simulink model "Parallel_n25_D2"  (R2012b)
settings: Solver=VariableStepDiscrete  StartTime=0.0  StopTime=TotalIterations  RelTol=1e-3
values from neighbouring files (symbols this model uses):
  bp = 12    [ConfigValidate.m]
  bpSNMemory = bp    (= 12)    [ConfigValidate.m]
  IterationsOrdering = 4000    [ConfigValidate.m]
  MaxCoordDistance = (abs(max(wx) - min(wx))+abs(max(wy) - min(wy)))^2    [ConfigValidate.m]
  N_limit = 0.01    [ConfigValidate.m]
  nBits = 9    [ConfigValidate.m]
  nBitsNSmemories = (ceil(log2(TotalIterations)))    [ConfigValidate.m]
  S_limit = 1    [ConfigValidate.m]
  SourceNodes = 2000    [ConfigValidate.m]
  ts = 1    [ConfigValidate.m]
  w1 = rand(1,Neurons)    [ConfigValidate.m]
  w2 = rand(1,Neurons)    [ConfigValidate.m]
  wx = zeros(1,Neurons)    [ConfigValidate.m]
  wy = zeros(1,Neurons)    [ConfigValidate.m]
  x1 = rand(SourceNodes,1)    [ConfigValidate.m]
  x2 = rand(SourceNodes,1)    [ConfigValidate.m]
libraries: xbsIndex_r4 x1652, dspsrcs4 x2, dspstat3 x2
(part 1 of 9)
settings Model: Creator=Leonardo  LastModifiedBy=leona

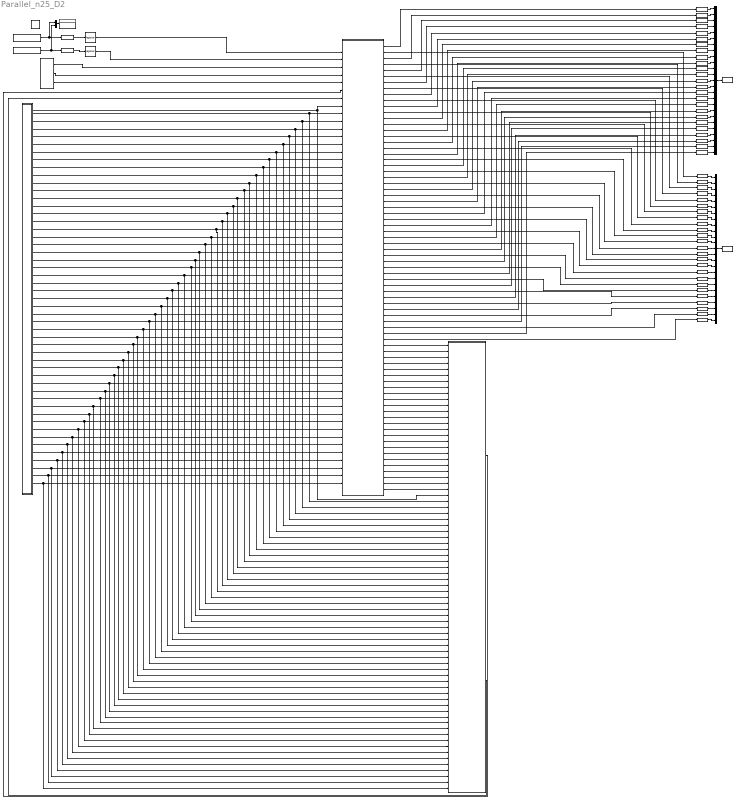
== system Parallel_n25_D2 ==
  " System Generator" : xbsIndex_r4/ System Generator  Tag=genX  xilinxfamily=virtex6  part=xc6vlx240t  speed=-1  package=ff1156  synthesis_tool=XST  clock_wrapper=Clock Enables  directory=./n25d2nt  proj_type=Project Navigator  Synth_file=XST Defaults  Impl_file=ISE Defaults  testbench=off  simulink_period=ts  sysclk_period=10  dcm_input_clock_period=10  incr_netlist=off  trim_vbits=Everywhere in SubSystem  dbl_ovrd=According to Block Masks  core_generation=According to Block Masks  run_coregen=off  deprecated_control=off  eval_field=0  block_type=sysgen
  Coordinates : Subsystem
  Display2 : Display
  Gateway Out{1..13,15..21,23..44,46..50} (47 alike) : xbsIndex_r4/Gateway Out  inherit_from_input=off  hdl_port=off  timing_constraint=None  locs_specified=off  LOCs={}  UseAsDAC=off  DACChannel='1'  block_type=gatewayout
  Gateway Out14 : xbsIndex_r4/Gateway Out  inherit_from_input=off  hdl_port=on  timing_constraint=None  locs_specified=off  LOCs={}  UseAsDAC=off  DACChannel='1'  block_type=gatewayout
  Gateway Out22 : xbsIndex_r4/Gateway Out  inherit_from_input=off  hdl_port=on  timing_constraint=None  locs_specified=off  LOCs={}  UseAsDAC=off  DACChannel='1'  block_type=gatewayout
  Gateway Out45 : xbsIndex_r4/Gateway Out  inherit_from_input=off  hdl_port=on  timing_constraint=None  locs_specified=off  LOCs={}  UseAsDAC=off  DACChannel='1'  block_type=gatewayout
  Mux3 : Mux  Inputs=2
  Mux5 : Mux  Inputs=25
  Mux6 : Mux  Inputs=25
  Neurons : Subsystem
  Signal From Workspace : dspsrcs4/Signal From Workspace  X=x1(1:SourceNodes)  Ts=ts  nsamps=1  OutputAfterFinalValue=Cyclic repetition  ignoreOrWarnInputAndFrameLengths=off
  Signal From Workspace1 : dspsrcs4/Signal From Workspace  X=x2(1:SourceNodes)  Ts=ts  nsamps=1  OutputAfterFinalValue=Cyclic repetition  ignoreOrWarnInputAndFrameLengths=off
  TimeSeries_Functions : Subsystem
  To Workspace : ToWorkspace  VariableName=w1_histH  SampleTime=ts
  To Workspace1 : ToWorkspace  VariableName=w2_histH  SampleTime=ts
  WiningNeuronFinder : Subsystem
  delay_vX11 : xbsIndex_r4/Register  init=x1(1)  rst=off  en=off  dbl_ovrd=off  block_type=register
  delay_vX12 : xbsIndex_r4/Register  init=x2(1)  rst=off  en=off  dbl_ovrd=off  block_type=register
  "vX11_in " : xbsIndex_r4/Gateway In  gui_display_data_type=Fixed-point  arith_type="Signed  (2's comp)"  n_bits=nb  bin_pt=bp  preci_type=Single  exp_width=8  frac_width=24  quantization="Round  (unbiased: +/- Inf)"  overflow=Saturate  period=ts  dbl_ovrd=off  timing_constraint=None  locs_specified=off  LOCs={}  UseAsADC=off  ADCChannel='1'  inherit_from_input=off  hdl_port=on  block_type=gatewayin
  vX12_in : xbsIndex_r4/Gateway In  gui_display_data_type=Fixed-point  arith_type="Signed  (2's comp)"  n_bits=nb  bin_pt=bp  preci_type=Single  exp_width=8  frac_width=24  quantization="Round  (unbiased: +/- Inf)"  overflow=Saturate  period=ts  dbl_ovrd=off  timing_constraint=None  locs_specified=off  LOCs={}  UseAsADC=off  ADCChannel='1'  inherit_from_input=off  hdl_port=on  block_type=gatewayin
  wires:
  Signal From Workspace/1 -> Mux3/1, "vX11_in "/1
  Signal From Workspace1/1 -> Mux3/2, vX12_in/1
  Mux3/1 -> Display2/1
  vX12_in/1 -> delay_vX12/1
  delay_vX12/1 -> Neurons/2(vX12)
  TimeSeries_Functions/1(S) -> Neurons/3(S)
  TimeSeries_Functions/2(N) -> Neurons/4(N)
  TimeSeries_Functions/3(MemControl) -> Neurons/5(memControl)
  Gateway Out1/1 -> Mux5/2
  Gateway Out14/1 -> Mux5/1
  Gateway Out10/1 -> Mux5/14
  Gateway Out8/1 -> Mux5/9
  Gateway Out17/1 -> Mux5/13
  Gateway Out6/1 -> Mux5/10
  Gateway Out4/1 -> Mux5/5
  Gateway Out2/1 -> Mux5/6
  Gateway Out13/1 -> Mux5/3
  Gateway Out15/1 -> Mux5/4
  Gateway Out9/1 -> Mux5/12
  Gateway Out18/1 -> Mux5/16
  Gateway Out7/1 -> Mux5/11
  Gateway Out16/1 -> Mux5/15
  Gateway Out3/1 -> Mux5/7
  Gateway Out5/1 -> Mux5/8
  Neurons/5(w1n3) -> Gateway Out13/1
  Neurons/7(w1n4) -> Gateway Out15/1
  Gateway Out19/1 -> Mux6/2
  Gateway Out22/1 -> Mux6/1
  Gateway Out20/1 -> Mux6/14
  Gateway Out33/1 -> Mux6/9
  Gateway Out25/1 -> Mux6/13
  Gateway Out31/1 -> Mux6/10
  Gateway Out29/1 -> Mux6/5
  Gateway Out27/1 -> Mux6/6
  Gateway Out21/1 -> Mux6/3
  Gateway Out23/1 -> Mux6/4
  Gateway Out34/1 -> Mux6/12
  Gateway Out26/1 -> Mux6/16
  Gateway Out32/1 -> Mux6/11
  Gateway Out24/1 -> Mux6/15
  Gateway Out28/1 -> Mux6/7
  Gateway Out30/1 -> Mux6/8
  Mux5/1 -> To Workspace/1
  Mux6/1 -> To Workspace1/1
  Neurons/53(dist_n3) -> WiningNeuronFinder/3(dist_k3)
  Neurons/52(dist_n2) -> WiningNeuronFinder/2(dist_k2)
  Neurons/54(dist_n4) -> WiningNeuronFinder/4(dist_k4)
  Neurons/51(dist_n1) -> WiningNeuronFinder/1(dist_k1)
  WiningNeuronFinder/1(WinningNeuron_wx) -> Neurons/6(wx_win)
  WiningNeuronFinder/2(WinningNeuron_wy) -> Neurons/7(wy_win)
  Neurons/55(dist_n5) -> WiningNeuronFinder/5(dist_k5)
  Neurons/56(dist_n6) -> WiningNeuronFinder/6(dist_k6)
  Neurons/57(dist_n7) -> WiningNeuronFinder/7(dist_k7)
  Neurons/58(dist_n8) -> WiningNeuronFinder/8(dist_k8)
  Neurons/59(dist_n9) -> WiningNeuronFinder/9(dist_k9)
  Neurons/60(dist_n10) -> WiningNeuronFinder/10(dist_k10)
  Neurons/61(dist_n11) -> WiningNeuronFinder/11(dist_k11)
  Neurons/62(dist_n12) -> WiningNeuronFinder/12(dist_k12)
  Neurons/63(dist_n13) -> WiningNeuronFinder/13(dist_k13)
  Neurons/64(dist_n14) -> WiningNeuronFinder/14(dist_k14)
  Neurons/65(dist_n15) -> WiningNeuronFinder/15(dist_k15)
  Neurons/66(dist_n16) -> WiningNeuronFinder/16(dist_k16)
  Neurons/67(dist_n17) -> WiningNeuronFinder/17(dist_k17)
  Neurons/68(dist_n18) -> WiningNeuronFinder/18(dist_k18)
  Neurons/69(dist_n19) -> WiningNeuronFinder/19(dist_k19)
  Neurons/70(dist_n20) -> WiningNeuronFinder/20(dist_k20)
  Neurons/71(dist_n21) -> WiningNeuronFinder/21(dist_k21)
  Neurons/72(dist_n22) -> WiningNeuronFinder/22(dist_k22)
  Neurons/73(dist_n23) -> WiningNeuronFinder/23(dist_k23)
  Neurons/74(dist_n24) -> WiningNeuronFinder/24(dist_k24)
  Neurons/75(dist_n25) -> WiningNeuronFinder/25(dist_k25)
  Coordinates/49(wx25) -> WiningNeuronFinder/74(wx_25), Neurons/56(wx25)
  Coordinates/48(wy24) -> WiningNeuronFinder/73(wy_24), Neurons/55(wy24)
  Coordinates/47(wx24) -> WiningNeuronFinder/72(wx_24), Neurons/54(wx24)
  Coordinates/46(wy23) -> WiningNeuronFinder/71(wy_23), Neurons/53(wy23)
  Coordinates/45(wx23) -> WiningNeuronFinder/70(wx_23), Neurons/52(wx23)
  Coordinates/44(wy22) -> WiningNeuronFinder/69(wy_22), Neurons/51(wy22)
  Coordinates/43(wx22) -> WiningNeuronFinder/68(wx_22), Neurons/50(wx22)
  Coordinates/42(wy21) -> WiningNeuronFinder/67(wy_21), Neurons/49(wy21)
  Coordinates/41(wx21) -> WiningNeuronFinder/66(wx_21), Neurons/48(wx21)
  Coordinates/40(wy20) -> WiningNeuronFinder/65(wy_20), Neurons/47(wy20)
  Coordinates/39(wx20) -> WiningNeuronFinder/64(wx_20), Neurons/46(wx20)
  Coordinates/38(wy19) -> WiningNeuronFinder/63(wy_19), Neurons/45(wy19)
  Coordinates/37(wx19) -> WiningNeuronFinder/62(wx_19), Neurons/44(wx19)
  Coordinates/36(wy18) -> WiningNeuronFinder/61(wy_18), Neurons/43(wy18)
  Coordinates/35(wx18) -> WiningNeuronFinder/60(wx_18), Neurons/42(wx18)
  Coordinates/34(wy17) -> WiningNeuronFinder/59(wy_17), Neurons/41(wy17)
  Coordinates/33(wx17) -> WiningNeuronFinder/58(wx_17), Neurons/40(wx17)
  Coordinates/32(wy16) -> WiningNeuronFinder/57(wy_16), Neurons/39(wy16)
  Coordinates/31(wx16) -> WiningNeuronFinder/56(wx_16), Neurons/38(wx16)
  Coordinates/30(wy15) -> WiningNeuronFinder/55(wy_15), Neurons/37(wy15)
  Coordinates/29(wx15) -> WiningNeuronFinder/54(wx_15), Neurons/36(wx15)
  Coordinates/28(wy14) -> WiningNeuronFinder/53(wy_14), Neurons/35(wy14)
  Coordinates/27(wx14) -> WiningNeuronFinder/52(wx_14), Neurons/34(wx14)
  Coordinates/25(wx13) -> WiningNeuronFinder/50(wx_13), Neurons/32(wx13)
  Coordinates/24(wy12) -> WiningNeuronFinder/49(wy_12), Neurons/31(wy12)
  Coordinates/23(wx12) -> WiningNeuronFinder/48(wx_12), Neurons/30(wx12)
  Coordinates/22(wy11) -> WiningNeuronFinder/47(wy_11), Neurons/29(wy11)
  Coordinates/21(wx11) -> WiningNeuronFinder/46(wx_11), Neurons/28(wx11)
  Coordinates/20(wy10) -> WiningNeuronFinder/45(wy_10), Neurons/27(wy10)
  Coordinates/19(wx10) -> WiningNeuronFinder/44(wx_10), Neurons/26(wx10)
  Coordinates/18(wy9) -> WiningNeuronFinder/43(wy_9), Neurons/25(wy9)
  Coordinates/17(wx9) -> WiningNeuronFinder/42(wx_9), Neurons/24(wx9)
  Coordinates/16(wy8) -> WiningNeuronFinder/41(wy_8), Neurons/23(wy8)
  Coordinates/15(wx8) -> WiningNeuronFinder/40(wx_8), Neurons/22(wx8)
  Coordinates/13(wx7) -> WiningNeuronFinder/38(wx_7), Neurons/20(wx7)
  Coordinates/12(wy6) -> WiningNeuronFinder/37(wy_6), Neurons/19(wy6)
  Coordinates/11(wx6) -> WiningNeuronFinder/36(wx_6), Neurons/18(wx6)
  Coordinates/10(wy5) -> WiningNeuronFinder/35(wy_5), Neurons/17(wy5)
  Coordinates/9(wx5) -> WiningNeuronFinder/34(wx_5), Neurons/16(wx5)
  Coordinates/8(wy4) -> WiningNeuronFinder/33(wy_4), Neurons/15(wy4)
  Coordinates/7(wx4) -> WiningNeuronFinder/32(wx_4), Neurons/14(wx4)
  Coordinates/6(wy3) -> WiningNeuronFinder/31(wy_3), Neurons/13(wy3)
  Coordinates/5(wx3) -> WiningNeuronFinder/30(wx_3), Neurons/12(wx3)
  Coordinates/4(wy2) -> WiningNeuronFinder/29(wy_2), Neurons/11(wy2)
  Coordinates/3(wx2) -> WiningNeuronFinder/28(wx_2), Neurons/10(wx2)
  Coordinates/2(wy1) -> WiningNeuronFinder/27(wy_1), Neurons/9(wy1)
  Coordinates/1(wx1) -> Neurons/8(wx1), WiningNeuronFinder/26(wx_1)
  Coordinates/14(wy7) -> WiningNeuronFinder/39(wy_7), Neurons/21(wy7)
  Coordinates/26(wy13) -> WiningNeuronFinder/51(wy_13), Neurons/33(wy13)
  Coordinates/50(wy25) -> WiningNeuronFinder/75(wy_25), Neurons/57(wy25)
  Neurons/9(w1n5) -> Gateway Out4/1
  Neurons/11(w1n6) -> Gateway Out2/1
  Neurons/13(w1n7) -> Gateway Out3/1
  Neurons/15(w1n8) -> Gateway Out5/1
  Neurons/17(w1n9) -> Gateway Out8/1
  Neurons/19(w1n10) -> Gateway Out6/1
  Neurons/21(w1n11) -> Gateway Out7/1
  Neurons/23(w1n12) -> Gateway Out9/1
  Neurons/25(w1n13) -> Gateway Out17/1
  Neurons/27(w1n14) -> Gateway Out10/1
  Neurons/29(w1n15) -> Gateway Out16/1
  Neurons/31(w1n16) -> Gateway Out18/1
  Gateway Out12/1 -> Mux5/24
  Gateway Out36/1 -> Mux5/25
  Gateway Out37/1 -> Mux5/17
  Gateway Out39/1 -> Mux5/20
  Gateway Out41/1 -> Mux5/21
  Gateway Out11/1 -> Mux5/23
  Gateway Out40/1 -> Mux5/18
  Gateway Out38/1 -> Mux5/19
  Gateway Out35/1 -> Mux5/22
  Neurons/33(w1n17) -> Gateway Out37/1
  Neurons/35(w1n18) -> Gateway Out40/1
  Neurons/37(w1n19) -> Gateway Out38/1
  Neurons/39(w1n20) -> Gateway Out39/1
  Neurons/41(w1n21) -> Gateway Out41/1
  Neurons/43(w1n22) -> Gateway Out35/1
  Neurons/45(w1n23) -> Gateway Out11/1
  Neurons/47(w1n24) -> Gateway Out12/1
  Neurons/49(w1n25) -> Gateway Out36/1
  Gateway Out43/1 -> Mux6/24
  Gateway Out46/1 -> Mux6/17
  Gateway Out50/1 -> Mux6/21
  Gateway Out48/1 -> Mux6/20
  Gateway Out45/1 -> Mux6/25
  Gateway Out42/1 -> Mux6/23
  Gateway Out44/1 -> Mux6/22
  Gateway Out49/1 -> Mux6/18
  Gateway Out47/1 -> Mux6/19
  Neurons/4(w2n2) -> Gateway Out19/1
  Neurons/6(w2n3) -> Gateway Out21/1
  Neurons/8(w2n4) -> Gateway Out23/1
  Neurons/10(w2n5) -> Gateway Out29/1
  Neurons/12(w2n6) -> Gateway Out27/1
  Neurons/14(w2n7) -> Gateway Out28/1
  Neurons/16(w2n8) -> Gateway Out30/1
  Neurons/18(w2n9) -> Gateway Out33/1
  Neurons/20(w2n10) -> Gateway Out31/1
  Neurons/22(w2n11) -> Gateway Out32/1
  Neurons/24(w2n12) -> Gateway Out34/1
  Neurons/26(w2n13) -> Gateway Out25/1
  Neurons/28(w2n14) -> Gateway Out20/1
  Neurons/30(w2n15) -> Gateway Out24/1
  Neurons/32(w2n16) -> Gateway Out26/1
  Neurons/34(w2n17) -> Gateway Out46/1
  Neurons/36(w2n18) -> Gateway Out49/1
  Neurons/38(w2n19) -> Gateway Out47/1
  Neurons/40(w2n20) -> Gateway Out48/1
  Neurons/42(w2n21) -> Gateway Out50/1
  Neurons/44(w2n22) -> Gateway Out44/1
  Neurons/46(w2n23) -> Gateway Out42/1
  Neurons/48(w2n24) -> Gateway Out43/1
  Neurons/50(w2n25) -> Gateway Out45/1
  "vX11_in "/1 -> delay_vX11/1
  delay_vX11/1 -> Neurons/1(vX11)
  Neurons/3(w1n2) -> Gateway Out1/1
  Neurons/1(w1n1) -> Gateway Out14/1
  Neurons/2(w2n1) -> Gateway Out22/1

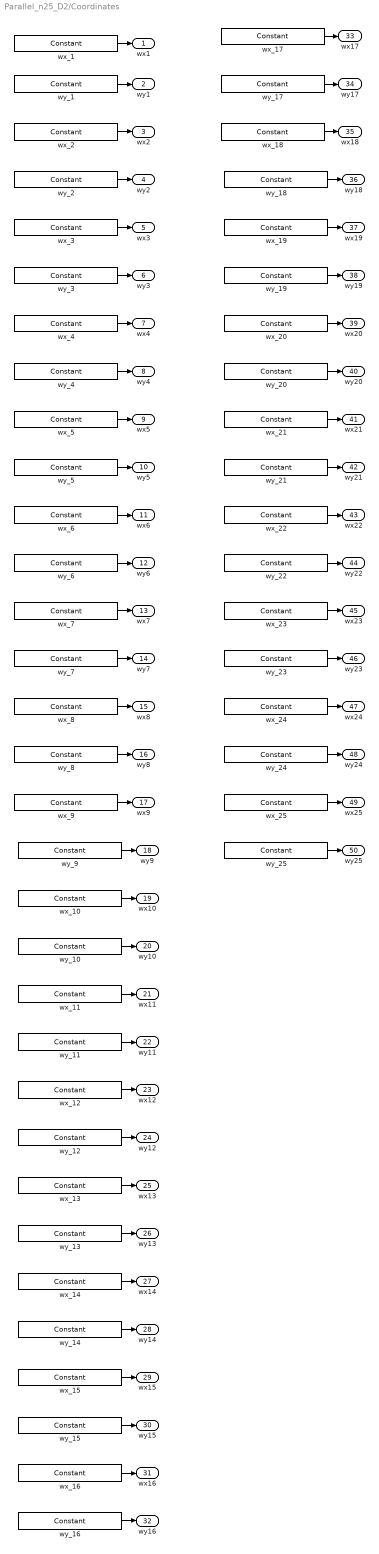
== system Parallel_n25_D2/Coordinates ==
  wx_1 : xbsIndex_r4/Constant  const=wx(1)  gui_display_data_type=Fixed-point  arith_type=Unsigned  n_bits=nbCoord  bin_pt=bpCoord  preci_type=Single  exp_width=8  frac_width=24  explicit_period=on  period=ts  equ=P=C  opselect=C  inp2=PCIN>>17  opr=+  inp1=P  carry=CIN  dbl_ovrd=off  block_type=constant
  wx_10 : xbsIndex_r4/Constant  const=wx(10)  gui_display_data_type=Fixed-point  arith_type=Unsigned  n_bits=nbCoord  bin_pt=bpCoord  preci_type=Single  exp_width=8  frac_width=24  explicit_period=on  period=ts  equ=P=C  opselect=C  inp2=PCIN>>17  opr=+  inp1=P  carry=CIN  dbl_ovrd=off  block_type=constant
  wx_11 : xbsIndex_r4/Constant  const=wx(11)  gui_display_data_type=Fixed-point  arith_type=Unsigned  n_bits=nbCoord  bin_pt=bpCoord  preci_type=Single  exp_width=8  frac_width=24  explicit_period=on  period=ts  equ=P=C  opselect=C  inp2=PCIN>>17  opr=+  inp1=P  carry=CIN  dbl_ovrd=off  block_type=constant
  wx_12 : xbsIndex_r4/Constant  const=wx(12)  gui_display_data_type=Fixed-point  arith_type=Unsigned  n_bits=nbCoord  bin_pt=bpCoord  preci_type=Single  exp_width=8  frac_width=24  explicit_period=on  period=ts  equ=P=C  opselect=C  inp2=PCIN>>17  opr=+  inp1=P  carry=CIN  dbl_ovrd=off  block_type=constant
  wx_13 : xbsIndex_r4/Constant  const=wx(13)  gui_display_data_type=Fixed-point  arith_type=Unsigned  n_bits=nbCoord  bin_pt=bpCoord  preci_type=Single  exp_width=8  frac_width=24  explicit_period=on  period=ts  equ=P=C  opselect=C  inp2=PCIN>>17  opr=+  inp1=P  carry=CIN  dbl_ovrd=off  block_type=constant
  wx_14 : xbsIndex_r4/Constant  const=wx(14)  gui_display_data_type=Fixed-point  arith_type=Unsigned  n_bits=nbCoord  bin_pt=bpCoord  preci_type=Single  exp_width=8  frac_width=24  explicit_period=on  period=ts  equ=P=C  opselect=C  inp2=PCIN>>17  opr=+  inp1=P  carry=CIN  dbl_ovrd=off  block_type=constant
  wx_15 : xbsIndex_r4/Constant  const=wx(15)  gui_display_data_type=Fixed-point  arith_type=Unsigned  n_bits=nbCoord  bin_pt=bpCoord  preci_type=Single  exp_width=8  frac_width=24  explicit_period=on  period=ts  equ=P=C  opselect=C  inp2=PCIN>>17  opr=+  inp1=P  carry=CIN  dbl_ovrd=off  block_type=constant
  wx_16 : xbsIndex_r4/Constant  const=wx(16)  gui_display_data_type=Fixed-point  arith_type=Unsigned  n_bits=nbCoord  bin_pt=bpCoord  preci_type=Single  exp_width=8  frac_width=24  explicit_period=on  period=ts  equ=P=C  opselect=C  inp2=PCIN>>17  opr=+  inp1=P  carry=CIN  dbl_ovrd=off  block_type=constant
  wx_17 : xbsIndex_r4/Constant  const=wx(17)  gui_display_data_type=Fixed-point  arith_type=Unsigned  n_bits=nbCoord  bin_pt=bpCoord  preci_type=Single  exp_width=8  frac_width=24  explicit_period=on  period=ts  equ=P=C  opselect=C  inp2=PCIN>>17  opr=+  inp1=P  carry=CIN  dbl_ovrd=off  block_type=constant
  wx_18 : xbsIndex_r4/Constant  const=wx(18)  gui_display_data_type=Fixed-point  arith_type=Unsigned  n_bits=nbCoord  bin_pt=bpCoord  preci_type=Single  exp_width=8  frac_width=24  explicit_period=on  period=ts  equ=P=C  opselect=C  inp2=PCIN>>17  opr=+  inp1=P  carry=CIN  dbl_ovrd=off  block_type=constant
  wx_19 : xbsIndex_r4/Constant  const=wx(19)  gui_display_data_type=Fixed-point  arith_type=Unsigned  n_bits=nbCoord  bin_pt=bpCoord  preci_type=Single  exp_width=8  frac_width=24  explicit_period=on  period=ts  equ=P=C  opselect=C  inp2=PCIN>>17  opr=+  inp1=P  carry=CIN  dbl_ovrd=off  block_type=constant
  wx_2 : xbsIndex_r4/Constant  const=wx(2)  gui_display_data_type=Fixed-point  arith_type=Unsigned  n_bits=nbCoord  bin_pt=bpCoord  preci_type=Single  exp_width=8  frac_width=24  explicit_period=on  period=ts  equ=P=C  opselect=C  inp2=PCIN>>17  opr=+  inp1=P  carry=CIN  dbl_ovrd=off  block_type=constant
  wx_20 : xbsIndex_r4/Constant  const=wx(20)  gui_display_data_type=Fixed-point  arith_type=Unsigned  n_bits=nbCoord  bin_pt=bpCoord  preci_type=Single  exp_width=8  frac_width=24  explicit_period=on  period=ts  equ=P=C  opselect=C  inp2=PCIN>>17  opr=+  inp1=P  carry=CIN  dbl_ovrd=off  block_type=constant
  wx_21 : xbsIndex_r4/Constant  const=wx(21)  gui_display_data_type=Fixed-point  arith_type=Unsigned  n_bits=nbCoord  bin_pt=bpCoord  preci_type=Single  exp_width=8  frac_width=24  explicit_period=on  period=ts  equ=P=C  opselect=C  inp2=PCIN>>17  opr=+  inp1=P  carry=CIN  dbl_ovrd=off  block_type=constant
  wx_22 : xbsIndex_r4/Constant  const=wx(22)  gui_display_data_type=Fixed-point  arith_type=Unsigned  n_bits=nbCoord  bin_pt=bpCoord  preci_type=Single  exp_width=8  frac_width=24  explicit_period=on  period=ts  equ=P=C  opselect=C  inp2=PCIN>>17  opr=+  inp1=P  carry=CIN  dbl_ovrd=off  block_type=constant
  wx_23 : xbsIndex_r4/Constant  const=wx(23)  gui_display_data_type=Fixed-point  arith_type=Unsigned  n_bits=nbCoord  bin_pt=bpCoord  preci_type=Single  exp_width=8  frac_width=24  explicit_period=on  period=ts  equ=P=C  opselect=C  inp2=PCIN>>17  opr=+  inp1=P  carry=CIN  dbl_ovrd=off  block_type=constant
  wx_24 : xbsIndex_r4/Constant  const=wx(24)  gui_display_data_type=Fixed-point  arith_type=Unsigned  n_bits=nbCoord  bin_pt=bpCoord  preci_type=Single  exp_width=8  frac_width=24  explicit_period=on  period=ts  equ=P=C  opselect=C  inp2=PCIN>>17  opr=+  inp1=P  carry=CIN  dbl_ovrd=off  block_type=constant
  wx_25 : xbsIndex_r4/Constant  const=wx(25)  gui_display_data_type=Fixed-point  arith_type=Unsigned  n_bits=nbCoord  bin_pt=bpCoord  preci_type=Single  exp_width=8  frac_width=24  explicit_period=on  period=ts  equ=P=C  opselect=C  inp2=PCIN>>17  opr=+  inp1=P  carry=CIN  dbl_ovrd=off  block_type=constant
  wx_3 : xbsIndex_r4/Constant  const=wx(3)  gui_display_data_type=Fixed-point  arith_type=Unsigned  n_bits=nbCoord  bin_pt=bpCoord  preci_type=Single  exp_width=8  frac_width=24  explicit_period=on  period=ts  equ=P=C  opselect=C  inp2=PCIN>>17  opr=+  inp1=P  carry=CIN  dbl_ovrd=off  block_type=constant
  wx_4 : xbsIndex_r4/Constant  const=wx(4)  gui_display_data_type=Fixed-point  arith_type=Unsigned  n_bits=nbCoord  bin_pt=bpCoord  preci_type=Single  exp_width=8  frac_width=24  explicit_period=on  period=ts  equ=P=C  opselect=C  inp2=PCIN>>17  opr=+  inp1=P  carry=CIN  dbl_ovrd=off  block_type=constant
  wx_5 : xbsIndex_r4/Constant  const=wx(5)  gui_display_data_type=Fixed-point  arith_type=Unsigned  n_bits=nbCoord  bin_pt=bpCoord  preci_type=Single  exp_width=8  frac_width=24  explicit_period=on  period=ts  equ=P=C  opselect=C  inp2=PCIN>>17  opr=+  inp1=P  carry=CIN  dbl_ovrd=off  block_type=constant
  wx_6 : xbsIndex_r4/Constant  const=wx(6)  gui_display_data_type=Fixed-point  arith_type=Unsigned  n_bits=nbCoord  bin_pt=bpCoord  preci_type=Single  exp_width=8  frac_width=24  explicit_period=on  period=ts  equ=P=C  opselect=C  inp2=PCIN>>17  opr=+  inp1=P  carry=CIN  dbl_ovrd=off  block_type=constant
  wx_7 : xbsIndex_r4/Constant  const=wx(7)  gui_display_data_type=Fixed-point  arith_type=Unsigned  n_bits=nbCoord  bin_pt=bpCoord  preci_type=Single  exp_width=8  frac_width=24  explicit_period=on  period=ts  equ=P=C  opselect=C  inp2=PCIN>>17  opr=+  inp1=P  carry=CIN  dbl_ovrd=off  block_type=constant
  wx_8 : xbsIndex_r4/Constant  const=wx(8)  gui_display_data_type=Fixed-point  arith_type=Unsigned  n_bits=nbCoord  bin_pt=bpCoord  preci_type=Single  exp_width=8  frac_width=24  explicit_period=on  period=ts  equ=P=C  opselect=C  inp2=PCIN>>17  opr=+  inp1=P  carry=CIN  dbl_ovrd=off  block_type=constant
  wx_9 : xbsIndex_r4/Constant  const=wx(9)  gui_display_data_type=Fixed-point  arith_type=Unsigned  n_bits=nbCoord  bin_pt=bpCoord  preci_type=Single  exp_width=8  frac_width=24  explicit_period=on  period=ts  equ=P=C  opselect=C  inp2=PCIN>>17  opr=+  inp1=P  carry=CIN  dbl_ovrd=off  block_type=constant
  wy_1 : xbsIndex_r4/Constant  const=wy(1)  gui_display_data_type=Fixed-point  arith_type=Unsigned  n_bits=nbCoord  bin_pt=bpCoord  preci_type=Single  exp_width=8  frac_width=24  explicit_period=on  period=ts  equ=P=C  opselect=C  inp2=PCIN>>17  opr=+  inp1=P  carry=CIN  dbl_ovrd=off  block_type=constant
  wy_10 : xbsIndex_r4/Constant  const=wy(10)  gui_display_data_type=Fixed-point  arith_type=Unsigned  n_bits=nbCoord  bin_pt=bpCoord  preci_type=Single  exp_width=8  frac_width=24  explicit_period=on  period=ts  equ=P=C  opselect=C  inp2=PCIN>>17  opr=+  inp1=P  carry=CIN  dbl_ovrd=off  block_type=constant
  wy_11 : xbsIndex_r4/Constant  const=wy(11)  gui_display_data_type=Fixed-point  arith_type=Unsigned  n_bits=nbCoord  bin_pt=bpCoord  preci_type=Single  exp_width=8  frac_width=24  explicit_period=on  period=ts  equ=P=C  opselect=C  inp2=PCIN>>17  opr=+  inp1=P  carry=CIN  dbl_ovrd=off  block_type=constant
  wy_12 : xbsIndex_r4/Constant  const=wy(12)  gui_display_data_type=Fixed-point  arith_type=Unsigned  n_bits=nbCoord  bin_pt=bpCoord  preci_type=Single  exp_width=8  frac_width=24  explicit_period=on  period=ts  equ=P=C  opselect=C  inp2=PCIN>>17  opr=+  inp1=P  carry=CIN  dbl_ovrd=off  block_type=constant
  wy_13 : xbsIndex_r4/Constant  const=wy(13)  gui_display_data_type=Fixed-point  arith_type=Unsigned  n_bits=nbCoord  bin_pt=bpCoord  preci_type=Single  exp_width=8  frac_width=24  explicit_period=on  period=ts  equ=P=C  opselect=C  inp2=PCIN>>17  opr=+  inp1=P  carry=CIN  dbl_ovrd=off  block_type=constant
  wy_14 : xbsIndex_r4/Constant  const=wy(14)  gui_display_data_type=Fixed-point  arith_type=Unsigned  n_bits=nbCoord  bin_pt=bpCoord  preci_type=Single  exp_width=8  frac_width=24  explicit_period=on  period=ts  equ=P=C  opselect=C  inp2=PCIN>>17  opr=+  inp1=P  carry=CIN  dbl_ovrd=off  block_type=constant
  wy_15 : xbsIndex_r4/Constant  const=wy(15)  gui_display_data_type=Fixed-point  arith_type=Unsigned  n_bits=nbCoord  bin_pt=bpCoord  preci_type=Single  exp_width=8  frac_width=24  explicit_period=on  period=ts  equ=P=C  opselect=C  inp2=PCIN>>17  opr=+  inp1=P  carry=CIN  dbl_ovrd=off  block_type=constant
  wy_16 : xbsIndex_r4/Constant  const=wy(16)  gui_display_data_type=Fixed-point  arith_type=Unsigned  n_bits=nbCoord  bin_pt=bpCoord  preci_type=Single  exp_width=8  frac_width=24  explicit_period=on  period=ts  equ=P=C  opselect=C  inp2=PCIN>>17  opr=+  inp1=P  carry=CIN  dbl_ovrd=off  block_type=constant
  wy_17 : xbsIndex_r4/Constant  const=wy(17)  gui_display_data_type=Fixed-point  arith_type=Unsigned  n_bits=nbCoord  bin_pt=bpCoord  preci_type=Single  exp_width=8  frac_width=24  explicit_period=on  period=ts  equ=P=C  opselect=C  inp2=PCIN>>17  opr=+  inp1=P  carry=CIN  dbl_ovrd=off  block_type=constant
  wy_18 : xbsIndex_r4/Constant  const=wy(18)  gui_display_data_type=Fixed-point  arith_type=Unsigned  n_bits=nbCoord  bin_pt=bpCoord  preci_type=Single  exp_width=8  frac_width=24  explicit_period=on  period=ts  equ=P=C  opselect=C  inp2=PCIN>>17  opr=+  inp1=P  carry=CIN  dbl_ovrd=off  block_type=constant
  wy_19 : xbsIndex_r4/Constant  const=wy(19)  gui_display_data_type=Fixed-point  arith_type=Unsigned  n_bits=nbCoord  bin_pt=bpCoord  preci_type=Single  exp_width=8  frac_width=24  explicit_period=on  period=ts  equ=P=C  opselect=C  inp2=PCIN>>17  opr=+  inp1=P  carry=CIN  dbl_ovrd=off  block_type=constant
  wy_2 : xbsIndex_r4/Constant  const=wy(2)  gui_display_data_type=Fixed-point  arith_type=Unsigned  n_bits=nbCoord  bin_pt=bpCoord  preci_type=Single  exp_width=8  frac_width=24  explicit_period=on  period=ts  equ=P=C  opselect=C  inp2=PCIN>>17  opr=+  inp1=P  carry=CIN  dbl_ovrd=off  block_type=constant
  wy_20 : xbsIndex_r4/Constant  const=wy(20)  gui_display_data_type=Fixed-point  arith_type=Unsigned  n_bits=nbCoord  bin_pt=bpCoord  preci_type=Single  exp_width=8  frac_width=24  explicit_period=on  period=ts  equ=P=C  opselect=C  inp2=PCIN>>17  opr=+  inp1=P  carry=CIN  dbl_ovrd=off  block_type=constant
  wy_21 : xbsIndex_r4/Constant  const=wy(21)  gui_display_data_type=Fixed-point  arith_type=Unsigned  n_bits=nbCoord  bin_pt=bpCoord  preci_type=Single  exp_width=8  frac_width=24  explicit_period=on  period=ts  equ=P=C  opselect=C  inp2=PCIN>>17  opr=+  inp1=P  carry=CIN  dbl_ovrd=off  block_type=constant
  wy_22 : xbsIndex_r4/Constant  const=wy(22)  gui_display_data_type=Fixed-point  arith_type=Unsigned  n_bits=nbCoord  bin_pt=bpCoord  preci_type=Single  exp_width=8  frac_width=24  explicit_period=on  period=ts  equ=P=C  opselect=C  inp2=PCIN>>17  opr=+  inp1=P  carry=CIN  dbl_ovrd=off  block_type=constant
  wy_23 : xbsIndex_r4/Constant  const=wy(23)  gui_display_data_type=Fixed-point  arith_type=Unsigned  n_bits=nbCoord  bin_pt=bpCoord  preci_type=Single  exp_width=8  frac_width=24  explicit_period=on  period=ts  equ=P=C  opselect=C  inp2=PCIN>>17  opr=+  inp1=P  carry=CIN  dbl_ovrd=off  block_type=constant
  wy_24 : xbsIndex_r4/Constant  const=wy(24)  gui_display_data_type=Fixed-point  arith_type=Unsigned  n_bits=nbCoord  bin_pt=bpCoord  preci_type=Single  exp_width=8  frac_width=24  explicit_period=on  period=ts  equ=P=C  opselect=C  inp2=PCIN>>17  opr=+  inp1=P  carry=CIN  dbl_ovrd=off  block_type=constant
  wy_25 : xbsIndex_r4/Constant  const=wy(25)  gui_display_data_type=Fixed-point  arith_type=Unsigned  n_bits=nbCoord  bin_pt=bpCoord  preci_type=Single  exp_width=8  frac_width=24  explicit_period=on  period=ts  equ=P=C  opselect=C  inp2=PCIN>>17  opr=+  inp1=P  carry=CIN  dbl_ovrd=off  block_type=constant
  wy_3 : xbsIndex_r4/Constant  const=wy(3)  gui_display_data_type=Fixed-point  arith_type=Unsigned  n_bits=nbCoord  bin_pt=bpCoord  preci_type=Single  exp_width=8  frac_width=24  explicit_period=on  period=ts  equ=P=C  opselect=C  inp2=PCIN>>17  opr=+  inp1=P  carry=CIN  dbl_ovrd=off  block_type=constant
  wy_4 : xbsIndex_r4/Constant  const=wy(4)  gui_display_data_type=Fixed-point  arith_type=Unsigned  n_bits=nbCoord  bin_pt=bpCoord  preci_type=Single  exp_width=8  frac_width=24  explicit_period=on  period=ts  equ=P=C  opselect=C  inp2=PCIN>>17  opr=+  inp1=P  carry=CIN  dbl_ovrd=off  block_type=constant
  wy_5 : xbsIndex_r4/Constant  const=wy(5)  gui_display_data_type=Fixed-point  arith_type=Unsigned  n_bits=nbCoord  bin_pt=bpCoord  preci_type=Single  exp_width=8  frac_width=24  explicit_period=on  period=ts  equ=P=C  opselect=C  inp2=PCIN>>17  opr=+  inp1=P  carry=CIN  dbl_ovrd=off  block_type=constant
  wy_6 : xbsIndex_r4/Constant  const=wy(6)  gui_display_data_type=Fixed-point  arith_type=Unsigned  n_bits=nbCoord  bin_pt=bpCoord  preci_type=Single  exp_width=8  frac_width=24  explicit_period=on  period=ts  equ=P=C  opselect=C  inp2=PCIN>>17  opr=+  inp1=P  carry=CIN  dbl_ovrd=off  block_type=constant
  wy_7 : xbsIndex_r4/Constant  const=wy(7)  gui_display_data_type=Fixed-point  arith_type=Unsigned  n_bits=nbCoord  bin_pt=bpCoord  preci_type=Single  exp_width=8  frac_width=24  explicit_period=on  period=ts  equ=P=C  opselect=C  inp2=PCIN>>17  opr=+  inp1=P  carry=CIN  dbl_ovrd=off  block_type=constant
  wy_8 : xbsIndex_r4/Constant  const=wy(8)  gui_display_data_type=Fixed-point  arith_type=Unsigned  n_bits=nbCoord  bin_pt=bpCoord  preci_type=Single  exp_width=8  frac_width=24  explicit_period=on  period=ts  equ=P=C  opselect=C  inp2=PCIN>>17  opr=+  inp1=P  carry=CIN  dbl_ovrd=off  block_type=constant
  wy_9 : xbsIndex_r4/Constant  const=wy(9)  gui_display_data_type=Fixed-point  arith_type=Unsigned  n_bits=nbCoord  bin_pt=bpCoord  preci_type=Single  exp_width=8  frac_width=24  explicit_period=on  period=ts  equ=P=C  opselect=C  inp2=PCIN>>17  opr=+  inp1=P  carry=CIN  dbl_ovrd=off  block_type=constant
  wx1 : Outport
  wy1 : Outport  Port=2
  wx2 : Outport  Port=3
  wy2 : Outport  Port=4
  wx3 : Outport  Port=5
  wy3 : Outport  Port=6
  wx4 : Outport  Port=7
  wy4 : Outport  Port=8
  wx5 : Outport  Port=9
  wy5 : Outport  Port=10
  wx6 : Outport  Port=11
  wy6 : Outport  Port=12
  wx7 : Outport  Port=13
  wy7 : Outport  Port=14
  wx8 : Outport  Port=15
  wy8 : Outport  Port=16
  wx9 : Outport  Port=17
  wy9 : Outport  Port=18
  wx10 : Outport  Port=19
  wy10 : Outport  Port=20
  wx11 : Outport  Port=21
  wy11 : Outport  Port=22
  wx12 : Outport  Port=23
  wy12 : Outport  Port=24
  wx13 : Outport  Port=25
  wy13 : Outport  Port=26
  wx14 : Outport  Port=27
  wy14 : Outport  Port=28
  wx15 : Outport  Port=29
  wy15 : Outport  Port=30
  wx16 : Outport  Port=31
  wy16 : Outport  Port=32
  wx17 : Outport  Port=33
  wy17 : Outport  Port=34
  wx18 : Outport  Port=35
  wy18 : Outport  Port=36
  wx19 : Outport  Port=37
  wy19 : Outport  Port=38
  wx20 : Outport  Port=39
  wy20 : Outport  Port=40
  wx21 : Outport  Port=41
  wy21 : Outport  Port=42
  wx22 : Outport  Port=43
  wy22 : Outport  Port=44
  wx23 : Outport  Port=45
  wy23 : Outport  Port=46
  wx24 : Outport  Port=47
  wy24 : Outport  Port=48
  wx25 : Outport  Port=49
  wy25 : Outport  Port=50
  wires:
  wy_2/1 -> wy2/1
  wy_16/1 -> wy16/1
  wx_9/1 -> wx9/1
  wy_3/1 -> wy3/1
  wx_3/1 -> wx3/1
  wy_5/1 -> wy5/1
  wx_2/1 -> wx2/1
  wx_12/1 -> wx12/1
  wy_6/1 -> wy6/1
  wx_11/1 -> wx11/1
  wy_11/1 -> wy11/1
  wy_14/1 -> wy14/1
  wy_8/1 -> wy8/1
  wy_7/1 -> wy7/1
  wx_8/1 -> wx8/1
  wx_5/1 -> wx5/1
  wx_4/1 -> wx4/1
  wx_7/1 -> wx7/1
  wx_15/1 -> wx15/1
  wy_1/1 -> wy1/1
  wy_4/1 -> wy4/1
  wx_16/1 -> wx16/1
  wx_6/1 -> wx6/1
  wy_13/1 -> wy13/1
  wx_14/1 -> wx14/1
  wy_15/1 -> wy15/1
  wx_10/1 -> wx10/1
  wy_10/1 -> wy10/1
  wx_13/1 -> wx13/1
  wy_9/1 -> wy9/1
  wy_12/1 -> wy12/1
  wy_25/1 -> wy25/1
  wx_18/1 -> wx18/1
  wx_21/1 -> wx21/1
  wx_20/1 -> wx20/1
  wy_20/1 -> wy20/1
  wy_23/1 -> wy23/1
  wy_17/1 -> wy17/1
  wx_17/1 -> wx17/1
  wx_24/1 -> wx24/1
  wx_25/1 -> wx25/1
  wy_22/1 -> wy22/1
  wx_23/1 -> wx23/1
  wy_24/1 -> wy24/1
  wx_19/1 -> wx19/1
  wy_19/1 -> wy19/1
  wx_22/1 -> wx22/1
  wy_18/1 -> wy18/1
  wy_21/1 -> wy21/1
  wx_1/1 -> wx1/1

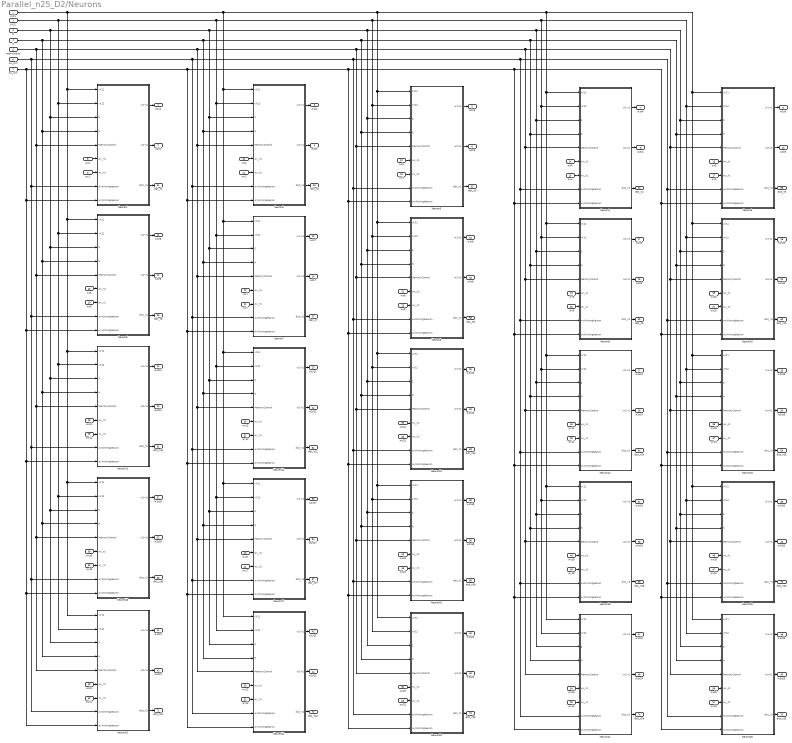
== system Parallel_n25_D2/Neurons ==
  vX11 : Inport
  vX12 : Inport  Port=2
  S : Inport  Port=3
  N : Inport  Port=4
  memControl : Inport  Port=5
  wx_win : Inport  Port=6
  wy_win : Inport  Port=7
  wx1 : Inport  Port=8
  wy1 : Inport  Port=9
  wx2 : Inport  Port=10
  wy2 : Inport  Port=11
  wx3 : Inport  Port=12
  wy3 : Inport  Port=13
  wx4 : Inport  Port=14
  wy4 : Inport  Port=15
  wx5 : Inport  Port=16
  wy5 : Inport  Port=17
  wx6 : Inport  Port=18
  wy6 : Inport  Port=19
  wx7 : Inport  Port=20
  wy7 : Inport  Port=21
  wx8 : Inport  Port=22
  wy8 : Inport  Port=23
  wx9 : Inport  Port=24
  wy9 : Inport  Port=25
  wx10 : Inport  Port=26
  wy10 : Inport  Port=27
  wx11 : Inport  Port=28
  wy11 : Inport  Port=29
  wx12 : Inport  Port=30
  wy12 : Inport  Port=31
  wx13 : Inport  Port=32
  wy13 : Inport  Port=33
  wx14 : Inport  Port=34
  wy14 : Inport  Port=35
  wx15 : Inport  Port=36
  wy15 : Inport  Port=37
  wx16 : Inport  Port=38
  wy16 : Inport  Port=39
  wx17 : Inport  Port=40
  wy17 : Inport  Port=41
  wx18 : Inport  Port=42
  wy18 : Inport  Port=43
  wx19 : Inport  Port=44
  wy19 : Inport  Port=45
  wx20 : Inport  Port=46
  wy20 : Inport  Port=47
  wx21 : Inport  Port=48
  wy21 : Inport  Port=49
  wx22 : Inport  Port=50
  wy22 : Inport  Port=51
  wx23 : Inport  Port=52
  wy23 : Inport  Port=53
  wx24 : Inport  Port=54
  wy24 : Inport  Port=55
  wx25 : Inport  Port=56
  wy25 : Inport  Port=57
  Neuron1 : Subsystem
  Neuron10 : Subsystem
  Neuron11 : Subsystem
  Neuron12 : Subsystem
  Neuron13 : Subsystem
  Neuron14 : Subsystem
  Neuron15 : Subsystem
  Neuron16 : Subsystem
  Neuron17 : Subsystem
  Neuron18 : Subsystem
  Neuron19 : Subsystem
  Neuron2 : Subsystem
  Neuron20 : Subsystem
  Neuron21 : Subsystem
  Neuron22 : Subsystem
  Neuron23 : Subsystem
  Neuron24 : Subsystem
  Neuron25 : Subsystem
  Neuron3 : Subsystem
  Neuron4 : Subsystem
  Neuron5 : Subsystem
  Neuron6 : Subsystem
  Neuron7 : Subsystem
  Neuron8 : Subsystem
  Neuron9 : Subsystem
  w1n1 : Outport
  w2n1 : Outport  Port=2
  w1n2 : Outport  Port=3
  w2n2 : Outport  Port=4
  w1n3 : Outport  Port=5
  w2n3 : Outport  Port=6
  w1n4 : Outport  Port=7
  w2n4 : Outport  Port=8
  w1n5 : Outport  Port=9
  w2n5 : Outport  Port=10
  w1n6 : Outport  Port=11
  w2n6 : Outport  Port=12
  w1n7 : Outport  Port=13
  w2n7 : Outport  Port=14
  w1n8 : Outport  Port=15
  w2n8 : Outport  Port=16
  w1n9 : Outport  Port=17
  w2n9 : Outport  Port=18
  w1n10 : Outport  Port=19
  w2n10 : Outport  Port=20
  w1n11 : Outport  Port=21
  w2n11 : Outport  Port=22
  w1n12 : Outport  Port=23
  w2n12 : Outport  Port=24
  w1n13 : Outport  Port=25
  w2n13 : Outport  Port=26
  w1n14 : Outport  Port=27
  w2n14 : Outport  Port=28
  w1n15 : Outport  Port=29
  w2n15 : Outport  Port=30
  w1n16 : Outport  Port=31
  w2n16 : Outport  Port=32
  w1n17 : Outport  Port=33
  w2n17 : Outport  Port=34
  w1n18 : Outport  Port=35
  w2n18 : Outport  Port=36
  w1n19 : Outport  Port=37
  w2n19 : Outport  Port=38
  w1n20 : Outport  Port=39
  w2n20 : Outport  Port=40
  w1n21 : Outport  Port=41
  w2n21 : Outport  Port=42
  w1n22 : Outport  Port=43
  w2n22 : Outport  Port=44
  w1n23 : Outport  Port=45
  w2n23 : Outport  Port=46
  w1n24 : Outport  Port=47
  w2n24 : Outport  Port=48
  w1n25 : Outport  Port=49
  w2n25 : Outport  Port=50
  dist_n1 : Outport  Port=51
  dist_n2 : Outport  Port=52
  dist_n3 : Outport  Port=53
  dist_n4 : Outport  Port=54
  dist_n5 : Outport  Port=55
  dist_n6 : Outport  Port=56
  dist_n7 : Outport  Port=57
  dist_n8 : Outport  Port=58
  dist_n9 : Outport  Port=59
  dist_n10 : Outport  Port=60
  dist_n11 : Outport  Port=61
  dist_n12 : Outport  Port=62
  dist_n13 : Outport  Port=63
  dist_n14 : Outport  Port=64
  dist_n15 : Outport  Port=65
  dist_n16 : Outport  Port=66
  dist_n17 : Outport  Port=67
  dist_n18 : Outport  Port=68
  dist_n19 : Outport  Port=69
  dist_n20 : Outport  Port=70
  dist_n21 : Outport  Port=71
  dist_n22 : Outport  Port=72
  dist_n23 : Outport  Port=73
  dist_n24 : Outport  Port=74
  dist_n25 : Outport  Port=75
  wires:
  wy1/1 -> Neuron1/7(wy_n1)
  Neuron2/1(w1-n1) -> w1n2/1
  Neuron3/2(w2-n1) -> w2n3/1
  Neuron1/1(w1-n1) -> w1n1/1
  Neuron2/2(w2-n1) -> w2n2/1
  Neuron1/2(w2-n1) -> w2n1/1
  wy3/1 -> Neuron3/7(wy_n1)
  wy2/1 -> Neuron2/7(wy_n1)
  Neuron3/1(w1-n1) -> w1n3/1
  wx3/1 -> Neuron3/6(wx_n1)
  wx2/1 -> Neuron2/6(wx_n1)
  Neuron4/2(w2-n1) -> w2n4/1
  wy4/1 -> Neuron4/7(wy_n1)
  wx4/1 -> Neuron4/6(wx_n1)
  Neuron4/1(w1-n1) -> w1n4/1
  Neuron1/3(dist_n1) -> dist_n1/1
  Neuron2/3(dist_n1) -> dist_n2/1
  Neuron3/3(dist_n1) -> dist_n3/1
  Neuron4/3(dist_n1) -> dist_n4/1
  memControl/1 -> Neuron5/5(MemoryControl), Neuron25/5(MemoryControl), Neuron20/5(MemoryControl), Neuron15/5(MemoryControl), Neuron10/5(MemoryControl), Neuron9/5(MemoryControl), Neuron24/5(MemoryControl), Neuron19/5(MemoryControl), Neuron14/5(MemoryControl), Neuron4/5(MemoryControl), Neuron23/5(MemoryControl), Neuron18/5(MemoryControl), Neuron13/5(MemoryControl), Neuron8/5(MemoryControl), Neuron3/5(MemoryControl), Neuron22/5(MemoryControl), Neuron17/5(MemoryControl), Neuron12/5(MemoryControl), Neuron7/5(MemoryControl), Neuron2/5(MemoryControl), Neuron21/5(MemoryControl), Neuron16/5(MemoryControl), Neuron11/5(MemoryControl), Neuron6/5(MemoryControl), Neuron1/5(MemoryControl)
  S/1 -> Neuron25/3(S), Neuron20/3(S), Neuron15/3(S), Neuron10/3(S), Neuron5/3(S), Neuron24/3(S), Neuron19/3(S), Neuron14/3(S), Neuron9/3(S), Neuron4/3(S), Neuron13/3(S), Neuron23/3(S), Neuron18/3(S), Neuron8/3(S), Neuron3/3(S), Neuron7/3(S), Neuron22/3(S), Neuron17/3(S), Neuron12/3(S), Neuron2/3(S), Neuron21/3(S), Neuron16/3(S), Neuron11/3(S), Neuron6/3(S), Neuron1/3(S)
  N/1 -> Neuron25/4(N), Neuron20/4(N), Neuron15/4(N), Neuron10/4(N), Neuron5/4(N), Neuron24/4(N), Neuron19/4(N), Neuron14/4(N), Neuron9/4(N), Neuron4/4(N), Neuron23/4(N), Neuron18/4(N), Neuron13/4(N), Neuron8/4(N), Neuron3/4(N), Neuron22/4(N), Neuron17/4(N), Neuron12/4(N), Neuron7/4(N), Neuron2/4(N), Neuron21/4(N), Neuron16/4(N), Neuron11/4(N), Neuron6/4(N), Neuron1/4(N)
  vX12/1 -> Neuron25/2(vX12), Neuron20/2(vX12), Neuron15/2(vX12), Neuron10/2(vX12), Neuron5/2(vX12), Neuron24/2(vX12), Neuron19/2(vX12), Neuron14/2(vX12), Neuron9/2(vX12), Neuron4/2(vX12), Neuron23/2(vX12), Neuron18/2(vX12), Neuron13/2(vX12), Neuron8/2(vX12), Neuron3/2(vX12), Neuron12/2(vX12), Neuron22/2(vX12), Neuron17/2(vX12), Neuron7/2(vX12), Neuron2/2(vX12), Neuron21/2(vX12), Neuron16/2(vX12), Neuron11/2(vX12), Neuron6/2(vX12), Neuron1/2(vX12)
  vX11/1 -> Neuron4/1(vX11), Neuron24/1(vX11), Neuron19/1(vX11), Neuron14/1(vX11), Neuron9/1(vX11), Neuron25/1(vX11), Neuron20/1(vX11), Neuron15/1(vX11), Neuron10/1(vX11), Neuron5/1(vX11), Neuron23/1(vX11), Neuron18/1(vX11), Neuron13/1(vX11), Neuron8/1(vX11), Neuron3/1(vX11), Neuron22/1(vX11), Neuron17/1(vX11), Neuron12/1(vX11), Neuron7/1(vX11), Neuron2/1(vX11), Neuron1/1(vX11), Neuron21/1(vX11), Neuron16/1(vX11), Neuron11/1(vX11), Neuron6/1(vX11)
  wx_win/1 -> Neuron24/8(wxWinningNeuron), Neuron19/8(wxWinningNeuron), Neuron14/8(wxWinningNeuron), Neuron9/8(wxWinningNeuron), Neuron4/8(wxWinningNeuron), Neuron25/8(wxWinningNeuron), Neuron20/8(wxWinningNeuron), Neuron15/8(wxWinningNeuron), Neuron10/8(wxWinningNeuron), Neuron5/8(wxWinningNeuron), Neuron23/8(wxWinningNeuron), Neuron18/8(wxWinningNeuron), Neuron13/8(wxWinningNeuron), Neuron8/8(wxWinningNeuron), Neuron3/8(wxWinningNeuron), Neuron22/8(wxWinningNeuron), Neuron17/8(wxWinningNeuron), Neuron12/8(wxWinningNeuron), Neuron7/8(wxWinningNeuron), Neuron2/8(wxWinningNeuron), Neuron21/8(wxWinningNeuron), Neuron16/8(wxWinningNeuron), Neuron11/8(wxWinningNeuron), Neuron6/8(wxWinningNeuron), Neuron1/8(wxWinningNeuron)
  wy_win/1 -> Neuron21/9(wyWinningNeuron), Neuron16/9(wyWinningNeuron), Neuron11/9(wyWinningNeuron), Neuron6/9(wyWinningNeuron), Neuron1/9(wyWinningNeuron), Neuron22/9(wyWinningNeuron), Neuron17/9(wyWinningNeuron), Neuron12/9(wyWinningNeuron), Neuron7/9(wyWinningNeuron), Neuron2/9(wyWinningNeuron), Neuron23/9(wyWinningNeuron), Neuron18/9(wyWinningNeuron), Neuron13/9(wyWinningNeuron), Neuron8/9(wyWinningNeuron), Neuron3/9(wyWinningNeuron), Neuron24/9(wyWinningNeuron), Neuron19/9(wyWinningNeuron), Neuron14/9(wyWinningNeuron), Neuron9/9(wyWinningNeuron), Neuron4/9(wyWinningNeuron), Neuron25/9(wyWinningNeuron), Neuron20/9(wyWinningNeuron), Neuron15/9(wyWinningNeuron), Neuron10/9(wyWinningNeuron), Neuron5/9(wyWinningNeuron)
  wy5/1 -> Neuron5/7(wy_n1)
  wx5/1 -> Neuron5/6(wx_n1)
  wy6/1 -> Neuron6/7(wy_n1)
  wx6/1 -> Neuron6/6(wx_n1)
  wy7/1 -> Neuron7/7(wy_n1)
  wx7/1 -> Neuron7/6(wx_n1)
  wy8/1 -> Neuron8/7(wy_n1)
  wx8/1 -> Neuron8/6(wx_n1)
  wy9/1 -> Neuron9/7(wy_n1)
  wx9/1 -> Neuron9/6(wx_n1)
  wy10/1 -> Neuron10/7(wy_n1)
  wx10/1 -> Neuron10/6(wx_n1)
  wy11/1 -> Neuron11/7(wy_n1)
  wx11/1 -> Neuron11/6(wx_n1)
  wy12/1 -> Neuron12/7(wy_n1)
  wx12/1 -> Neuron12/6(wx_n1)
  wy13/1 -> Neuron13/7(wy_n1)
  wx13/1 -> Neuron13/6(wx_n1)
  wy14/1 -> Neuron14/7(wy_n1)
  wx14/1 -> Neuron14/6(wx_n1)
  wy15/1 -> Neuron15/7(wy_n1)
  wx15/1 -> Neuron15/6(wx_n1)
  wy16/1 -> Neuron16/7(wy_n1)
  wx16/1 -> Neuron16/6(wx_n1)
  wy17/1 -> Neuron17/7(wy_n1)
  wx17/1 -> Neuron17/6(wx_n1)
  wy18/1 -> Neuron18/7(wy_n1)
  wx18/1 -> Neuron18/6(wx_n1)
  wy19/1 -> Neuron19/7(wy_n1)
  wx19/1 -> Neuron19/6(wx_n1)
  wy20/1 -> Neuron20/7(wy_n1)
  wx20/1 -> Neuron20/6(wx_n1)
  wy21/1 -> Neuron21/7(wy_n1)
  wx21/1 -> Neuron21/6(wx_n1)
  wy22/1 -> Neuron22/7(wy_n1)
  wx22/1 -> Neuron22/6(wx_n1)
  wy23/1 -> Neuron23/7(wy_n1)
  wx23/1 -> Neuron23/6(wx_n1)
  wy24/1 -> Neuron24/7(wy_n1)
  wx24/1 -> Neuron24/6(wx_n1)
  wy25/1 -> Neuron25/7(wy_n1)
  wx25/1 -> Neuron25/6(wx_n1)
  Neuron5/2(w2-n1) -> w2n5/1
  Neuron5/1(w1-n1) -> w1n5/1
  Neuron6/2(w2-n1) -> w2n6/1
  Neuron6/1(w1-n1) -> w1n6/1
  Neuron7/2(w2-n1) -> w2n7/1
  Neuron7/1(w1-n1) -> w1n7/1
  Neuron8/2(w2-n1) -> w2n8/1
  Neuron8/1(w1-n1) -> w1n8/1
  Neuron9/2(w2-n1) -> w2n9/1
  Neuron9/1(w1-n1) -> w1n9/1
  Neuron10/2(w2-n1) -> w2n10/1
  Neuron10/1(w1-n1) -> w1n10/1
  Neuron11/2(w2-n1) -> w2n11/1
  Neuron11/1(w1-n1) -> w1n11/1
  Neuron12/2(w2-n1) -> w2n12/1
  Neuron12/1(w1-n1) -> w1n12/1
  Neuron13/2(w2-n1) -> w2n13/1
  Neuron13/1(w1-n1) -> w1n13/1
  Neuron14/2(w2-n1) -> w2n14/1
  Neuron14/1(w1-n1) -> w1n14/1
  Neuron15/2(w2-n1) -> w2n15/1
  Neuron15/1(w1-n1) -> w1n15/1
  Neuron16/2(w2-n1) -> w2n16/1
  Neuron16/1(w1-n1) -> w1n16/1
  Neuron17/2(w2-n1) -> w2n17/1
  Neuron17/1(w1-n1) -> w1n17/1
  Neuron18/2(w2-n1) -> w2n18/1
  Neuron18/1(w1-n1) -> w1n18/1
  Neuron19/2(w2-n1) -> w2n19/1
  Neuron19/1(w1-n1) -> w1n19/1
  Neuron20/2(w2-n1) -> w2n20/1
  Neuron20/1(w1-n1) -> w1n20/1
  Neuron21/2(w2-n1) -> w2n21/1
  Neuron21/1(w1-n1) -> w1n21/1
  Neuron22/2(w2-n1) -> w2n22/1
  Neuron22/1(w1-n1) -> w1n22/1
  Neuron23/2(w2-n1) -> w2n23/1
  Neuron23/1(w1-n1) -> w1n23/1
  Neuron24/2(w2-n1) -> w2n24/1
  Neuron24/1(w1-n1) -> w1n24/1
  Neuron25/2(w2-n1) -> w2n25/1
  Neuron25/1(w1-n1) -> w1n25/1
  Neuron5/3(dist_n1) -> dist_n5/1
  Neuron6/3(dist_n1) -> dist_n6/1
  Neuron7/3(dist_n1) -> dist_n7/1
  Neuron8/3(dist_n1) -> dist_n8/1
  Neuron9/3(dist_n1) -> dist_n9/1
  Neuron10/3(dist_n1) -> dist_n10/1
  Neuron11/3(dist_n1) -> dist_n11/1
  Neuron12/3(dist_n1) -> dist_n12/1
  Neuron13/3(dist_n1) -> dist_n13/1
  Neuron14/3(dist_n1) -> dist_n14/1
  Neuron15/3(dist_n1) -> dist_n15/1
  Neuron16/3(dist_n1) -> dist_n16/1
  Neuron17/3(dist_n1) -> dist_n17/1
  Neuron18/3(dist_n1) -> dist_n18/1
  Neuron19/3(dist_n1) -> dist_n19/1
  Neuron20/3(dist_n1) -> dist_n20/1
  Neuron21/3(dist_n1) -> dist_n21/1
  Neuron22/3(dist_n1) -> dist_n22/1
  Neuron23/3(dist_n1) -> dist_n23/1
  Neuron24/3(dist_n1) -> dist_n24/1
  Neuron25/3(dist_n1) -> dist_n25/1
  wx1/1 -> Neuron1/6(wx_n1)

== system Parallel_n25_D2/TimeSeries_Functions ==
  note: Neighbor Function.
      | In the memory is stored the result of 1/2S² considering that S start from sqrt(neurons) and decrease to 1 (minimum value).
      | To avoid execute a divisor circuit inside the FPGA, in the memory is already stored the result of the division 1/2S² instead of stores only S
  note: Learning Function
      | The learning rate descreases from 0.1 to 0.001 during
      | ordering phase. In the covergence phase stays at the minimum.
  note: This circuits prevents all the memories in the circuit from working in the first clock cycle.
      | This helps prevent a response for a input equal to 1 in the beggining of the process.
  note: Note that the selector circuits in the memories are used to prevent the values
      | being less than the minimum value of each parameter during the ordering phase.
      | During the covergence phase it forces the minimum value
  Display{1..6} (6 alike) : Display
  DistMenor1 : xbsIndex_r4/Mux  inputs=2  en=off  latency=dMUX_CooperatingProcess  precision=Full  arith_type=Unsigned  n_bits=16  bin_pt=14  quantization=Truncate  overflow=Wrap  dbl_ovrd=off  block_type=mux
  DistMenor2 : xbsIndex_r4/Mux  inputs=2  en=off  latency=dMUX_CooperatingProcess  precision=Full  arith_type=Unsigned  n_bits=16  bin_pt=14  quantization=Truncate  overflow=Wrap  dbl_ovrd=off  block_type=mux
  Dist_compare1 : xbsIndex_r4/Relational  mode=a<=b  en=off  latency=dComparator_CooperatingProcess  dbl_ovrd=off  block_type=relational
  Dist_compare2 : xbsIndex_r4/Relational  mode=a>b  en=off  latency=dComparator_CooperatingProcess  dbl_ovrd=off  block_type=relational
  Dist_compare3 : xbsIndex_r4/Relational  mode=a>b  en=off  latency=dComparator_CooperatingProcess  dbl_ovrd=off  block_type=relational
  Dist_compare4 : xbsIndex_r4/Relational  mode=a=b  en=off  latency=dComparator_CooperatingProcess  dbl_ovrd=off  block_type=relational
  Gateway Out{1..6} (6 alike) : xbsIndex_r4/Gateway Out  inherit_from_input=off  hdl_port=off  timing_constraint=None  locs_specified=off  LOCs={}  UseAsDAC=off  DACChannel='1'  block_type=gatewayout
  Inverter : xbsIndex_r4/Inverter  en=off  latency=dInverter_CooperatingProcess  dbl_ovrd=off  block_type=inv
  LearningRateLimit : xbsIndex_r4/Constant  const=N_limit  gui_display_data_type=Fixed-point  arith_type=Signed (2's comp)  n_bits=bpSNMemory+1  bin_pt=bpSNMemory  preci_type=Single  exp_width=8  frac_width=24  explicit_period=on  period=ts  equ=P=C  opselect=C  inp2=PCIN>>17  opr=+  inp1=P  carry=CIN  dbl_ovrd=off  block_type=constant
  Learning_Rate : xbsIndex_r4/ROM  depth=2^nBitsNSmemories  initVector=N  distributed_mem=Block RAM  rst=off  init_reg=0  en=off  latency=dMemoryLearning  gui_display_data_type=Fixed-point  arith_type="Signed  (2's comp)"  n_bits=bpSNMemory+1  bin_pt=bpSNMemory  preci_type=Single  exp_width=8  frac_width=24  dbl_ovrd=off  optimize=Area  use_rpm=on  block_type=sprom
  Logical1 : xbsIndex_r4/Logical  logical_function=OR  inputs=2  en=off  latency=dOR_CooperatingProcess  precision=Full  arith_type=Unsigned  n_bits=16  bin_pt=0  align_bp=on  dbl_ovrd=off  block_type=logical
  Logical2 : xbsIndex_r4/Logical  logical_function=OR  inputs=2  en=off  latency=dOR_CooperatingProcess  precision=Full  arith_type=Unsigned  n_bits=16  bin_pt=0  align_bp=on  dbl_ovrd=off  block_type=logical
  Logical3 : xbsIndex_r4/Logical  logical_function=OR  inputs=2  en=off  latency=dAnd_CooperatingProcess  precision=Full  arith_type=Unsigned  n_bits=16  bin_pt=0  align_bp=on  dbl_ovrd=off  block_type=logical
  Neighborhood_Size : xbsIndex_r4/ROM  depth=2^nBitsNSmemories  initVector=S  distributed_mem=Block RAM  rst=off  init_reg=0  en=off  latency=dMemoryNeighbor  gui_display_data_type=Fixed-point  arith_type="Signed  (2's comp)"  n_bits=bpSNMemory+1  bin_pt=bpSNMemory  preci_type=Single  exp_width=8  frac_width=24  dbl_ovrd=off  optimize=Area  use_rpm=on  block_type=sprom
  Neighborhood_Size_Limit : xbsIndex_r4/Constant  const=S_limit  gui_display_data_type=Fixed-point  arith_type=Signed (2's comp)  n_bits=bpSNMemory+1  bin_pt=bpSNMemory  preci_type=Single  exp_width=8  frac_width=24  explicit_period=on  period=ts  equ=P=C  opselect=C  inp2=PCIN>>17  opr=+  inp1=P  carry=CIN  dbl_ovrd=off  block_type=constant
  OrderingPhase_offset : xbsIndex_r4/Constant  const=IterationsOrdering  gui_display_data_type=Fixed-point  arith_type=Unsigned  n_bits=12  bin_pt=0  preci_type=Single  exp_width=8  frac_width=24  explicit_period=on  period=ts  equ=P=C  opselect=C  inp2=PCIN>>17  opr=+  inp1=P  carry=CIN  dbl_ovrd=off  block_type=constant
  To Workspace : ToWorkspace  VariableName=S_histH  SampleTime=ts
  To Workspace1 : ToWorkspace  VariableName=N_histH  SampleTime=ts
  ZeroConstant : xbsIndex_r4/Constant  const=0  gui_display_data_type=Fixed-point  arith_type=Signed (2's comp)  n_bits=bpSNMemory+1  bin_pt=bpSNMemory  preci_type=Single  exp_width=8  frac_width=24  explicit_period=on  period=ts  equ=P=C  opselect=C  inp2=PCIN>>17  opr=+  inp1=P  carry=CIN  dbl_ovrd=off  block_type=constant
  count_reset : xbsIndex_r4/Counter  cnt_type=Free Running  cnt_to=(2^nBitsNSmemories)-1  operation=Up  start_count=0  cnt_by_val=1  arith_type=Unsigned  n_bits=nBitsNSmemories  bin_pt=0  load_pin=off  rst=off  en=on  explicit_period=on  period=ts  dbl_ovrd=off  use_behavioral_HDL=off  implementation=Fabric  block_type=counter
  delay_vX1 : xbsIndex_r4/Register  init=N_limit  rst=off  en=off  dbl_ovrd=off  block_type=register
  enable_bit : xbsIndex_r4/Constant  const=1  gui_display_data_type=Boolean  arith_type=Boolean  n_bits=nb  bin_pt=bp  preci_type=Single  exp_width=8  frac_width=24  explicit_period=on  period=ts  equ=P=C  opselect=C  inp2=PCIN>>17  opr=+  inp1=P  carry=CIN  dbl_ovrd=off  block_type=constant
  w1n1 : xbsIndex_r4/Register  init=0  rst=off  en=on  dbl_ovrd=off  block_type=register
  S : Outport
  N : Outport  Port=2
  MemControl : Outport  Port=3
  wires:
  w1n1/1 -> count_reset/1, MemControl/1, Inverter/1
  Inverter/1 -> w1n1/2
  enable_bit/1 -> w1n1/1
  DistMenor1/1 -> delay_vX1/1, Gateway Out6/1
  Gateway Out6/1 -> Display4/1, To Workspace1/1
  count_reset/1 -> Learning_Rate/1, Gateway Out4/1, Dist_compare3/1, Neighborhood_Size/1
  LearningRateLimit/1 -> DistMenor1/3, Dist_compare1/2
  Gateway Out5/1 -> To Workspace/1, Display3/1
  Neighborhood_Size/1 -> DistMenor2/2, Dist_compare2/1, Dist_compare4/1
  DistMenor2/1 -> S/1, Gateway Out5/1
  OrderingPhase_offset/1 -> Dist_compare3/2
  Dist_compare3/1 -> Logical1/1, Gateway Out1/1, Logical2/2
  Neighborhood_Size_Limit/1 -> DistMenor2/3, Dist_compare2/2
  Logical2/1 -> Gateway Out2/1, DistMenor2/1
  Logical1/1 -> Gateway Out3/1, DistMenor1/1
  Learning_Rate/1 -> DistMenor1/2, Dist_compare1/1
  Dist_compare1/1 -> Logical1/2
  Gateway Out1/1 -> Display1/1
  Gateway Out2/1 -> Display2/1
  Gateway Out3/1 -> Display5/1
  Gateway Out4/1 -> Display6/1
  Logical3/1 -> Logical2/1
  Dist_compare2/1 -> Logical3/2
  Dist_compare4/1 -> Logical3/1
  ZeroConstant/1 -> Dist_compare4/2
  delay_vX1/1 -> N/1
